simulink model "ragadozozsakmany"  (Simulink 7.7)
settings: Solver=ode3  StartTime=0.0  StopTime=20  FixedStep=0.01  RelTol=1e-3
settings Model: Creator=Rudi  LastModifiedBy=Rudi

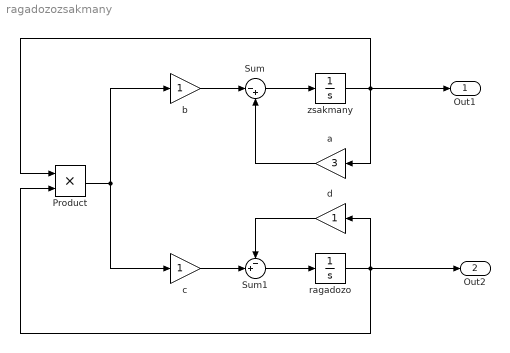
== system ragadozozsakmany ==
  Product : Product  RndMeth=Zero
  Sum : Sum  Inputs=|-+
  Sum1 : Sum  Inputs=-+|
  a : Gain  Gain=3
  b : Gain
  c : Gain
  d : Gain
  ragadozo : Integrator  InitialCondition=3
  zsakmany : Integrator  InitialCondition=2
  Out1 : Outport
  Out2 : Outport  Port=2
  wires:
  b/1 -> Sum/1
  ragadozo/1 -> d/1, Product/2, Out2/1
  d/1 -> Sum1/1
  c/1 -> Sum1/2
  Sum1/1 -> ragadozo/1
  zsakmany/1 -> a/1, Product/1, Out1/1
  a/1 -> Sum/2
  Sum/1 -> zsakmany/1
  Product/1 -> b/1, c/1
